simulink subsystem "Estimador_Estado_Reducido"  (R2026a)
settings: Solver=VariableStepAuto
values from neighbouring files (symbols this model uses):
  J_eq = J_m + J_l/(r_m2l^2)    (= 4.58263888889e-05)    [coeficientes.m]
  K_et = 1    [coeficientes.m]
  K_ew = 1    [coeficientes.m]
settings Model: Creator=admin  LastModifiedBy=admin

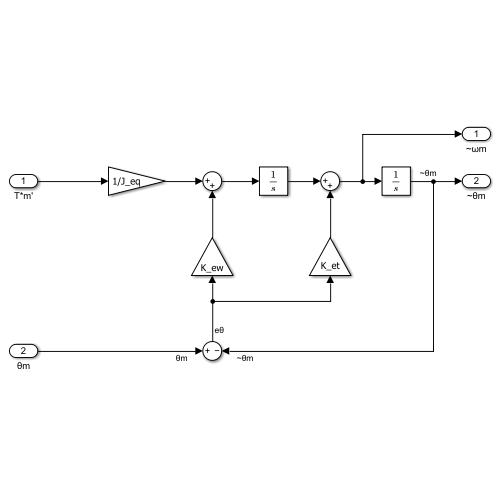
[thumbnail: Simulink's stored preview of the top-level diagram]
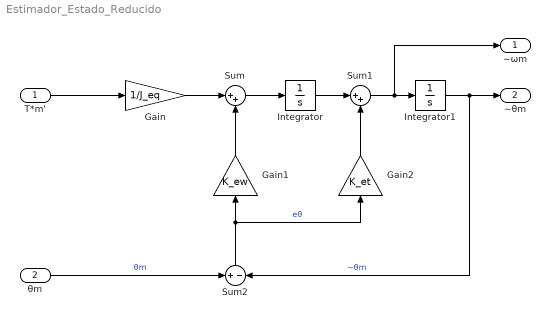
== system Estimador_Estado_Reducido ==
  T*m' : Inport
  θm : Inport  Port=2
  Gain : Gain  Gain=1/J_eq
  Gain1 : Gain  Gain=K_ew
  Gain2 : Gain  Gain=K_et
  Integrator : Integrator
  Integrator1 : Integrator
  Sum : Sum  Inputs=|++
  Sum1 : Sum  Inputs=|++
  Sum2 : Sum  Inputs=+-
  ~ωm : Outport
  ~θm : Outport  Port=2
  wires:
  T*m'/1 -> Gain/1
  Gain/1 -> Sum/1
  Sum/1 -> Integrator/1
  Sum1/1 -> ~ωm/1, Integrator1/1
  Integrator/1 -> Sum1/1
  Gain1/1 -> Sum/2
  Gain2/1 -> Sum1/2
  Sum2/1 -> Gain2/1, Gain1/1  "eθ"
  θm/1 -> Sum2/1  "θm"
  Integrator1/1 -> Sum2/2, ~θm/1  "~θm"
